simulink model "Q3n"  (R2018a)
settings: Solver=FixedStepDiscrete  StartTime=0.0  StopTime=0.42  RelTol=1e-3
libraries: powerlib x14, powerlib_meascontrol x3, dspstat3 x2, pePowerMeasurement x1
settings Model: Creator=hakkı  LastModifiedBy=hakkı

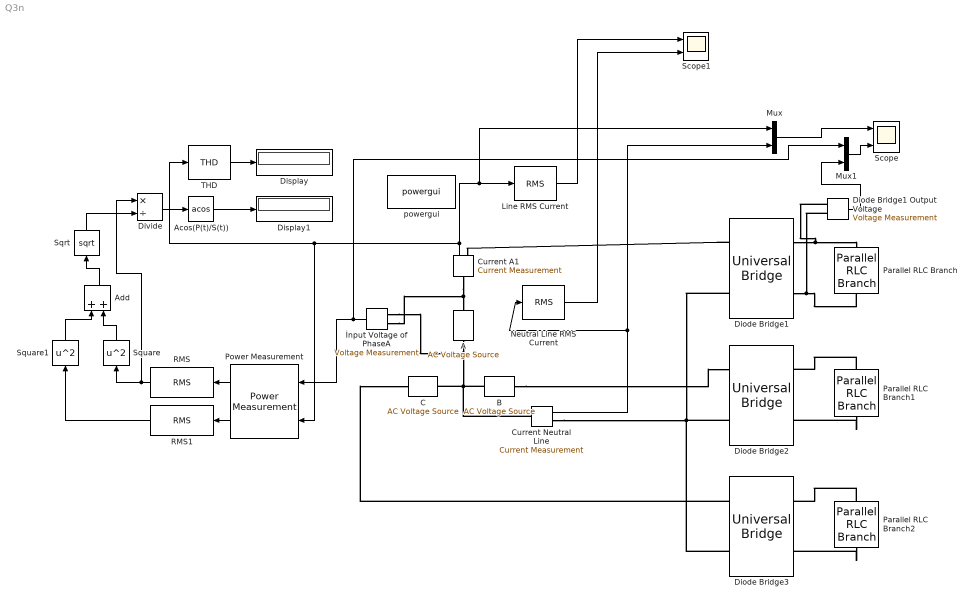
== system Q3n ==
  " İnput Voltage of PhaseA " : powerlib/Measurements/Voltage Measurement  PhasorSimulation=off  OutputType=Complex  PSBequivalent=0
  A : powerlib/Electrical Sources/AC Voltage Source  Amplitude=326.5986323710904130929712099607855189287929974208893504576  Phase=0  Frequency=50  SampleTime=0  Measurements=None  BusType=swing  Pref=10e3  Qref=0  Qmin=-inf  Qmax=+inf
  Acos(P(t)/S(t)) : Trigonometry  Operator=acos
  Add : Sum
  B : powerlib/Electrical Sources/AC Voltage Source  Amplitude=326.5986323710904130929712099607855189287929974208893504576  Phase=120  Frequency=50  SampleTime=0  Measurements=None  BusType=swing  Pref=10e3  Qref=0  Qmin=-inf  Qmax=+inf
  C : powerlib/Electrical Sources/AC Voltage Source  Amplitude=326.5986323710904130929712099607855189287929974208893504576  Phase=240  Frequency=50  SampleTime=0  Measurements=None  BusType=swing  Pref=10e3  Qref=0  Qmin=-inf  Qmax=+inf
  Current A1 : powerlib/Measurements/Current Measurement  PhasorSimulation=off  OutputType=Complex  PSBequivalent=0
  Current Neutral Line : powerlib/Measurements/Current Measurement  PhasorSimulation=off  OutputType=Complex  PSBequivalent=0
  Diode Bridge1 : powerlib/Power Electronics/Universal Bridge  Arms=2  SnubberResistance=1e5  SnubberCapacitance=inf  Device=Diodes  Ron=1e-3  Lon=0  ForwardVoltages="[  0  0  ]"  ForwardVoltage=0  GTOparameters=[ 10e-6 , 20e-6 ]  IGBTparameters=[ 1e-6 , 2e-6 ]  Measurements=None  Measurements_2=None  converterType=Rectifier
  "Diode Bridge1 Output Voltage " : powerlib/Measurements/Voltage Measurement  PhasorSimulation=off  OutputType=Complex  PSBequivalent=0
  Diode Bridge2 : powerlib/Power Electronics/Universal Bridge  Arms=2  SnubberResistance=1e5  SnubberCapacitance=inf  Device=Diodes  Ron=1e-3  Lon=0  ForwardVoltages="[  0  0  ]"  ForwardVoltage=0  GTOparameters=[ 10e-6 , 20e-6 ]  IGBTparameters=[ 1e-6 , 2e-6 ]  Measurements=None  Measurements_2=None  converterType=Rectifier
  Diode Bridge3 : powerlib/Power Electronics/Universal Bridge  Arms=2  SnubberResistance=1e5  SnubberCapacitance=inf  Device=Diodes  Ron=1e-3  Lon=0  ForwardVoltages="[  0  0  ]"  ForwardVoltage=0  GTOparameters=[ 10e-6 , 20e-6 ]  IGBTparameters=[ 1e-6 , 2e-6 ]  Measurements=None  Measurements_2=None  converterType=Rectifier
  Display : Display
  Display1 : Display
  Divide : Product  Inputs=*/
  "Line RMS Current " : powerlib_meascontrol/Measurements/RMS  TrueRMS=on  Freq=50  RMSInit=0  Ts=1e-6
  Mux : Mux  Inputs=2
  Mux1 : Mux  Inputs=2
  Neutral Line RMS Current : powerlib_meascontrol/Measurements/RMS  TrueRMS=on  Freq=50  RMSInit=0  Ts=1e-6
  Parallel RLC Branch : powerlib/Elements/Parallel RLC Branch  LConnTagsString=a  RConnTagsString=__new0  BranchType=RC  Resistance=200  Inductance=1e-3  SetiL0=off  InitialCurrent=0  Capacitance=470e-6  Setx0=off  InitialVoltage=0  Measurements=None
  Parallel RLC Branch1 : powerlib/Elements/Parallel RLC Branch  LConnTagsString=a  RConnTagsString=__new0  BranchType=RC  Resistance=200  Inductance=1e-3  SetiL0=off  InitialCurrent=0  Capacitance=470e-6  Setx0=off  InitialVoltage=0  Measurements=None
  Parallel RLC Branch2 : powerlib/Elements/Parallel RLC Branch  LConnTagsString=a  RConnTagsString=__new0  BranchType=RC  Resistance=200  Inductance=1e-3  SetiL0=off  InitialCurrent=0  Capacitance=470e-6  Setx0=off  InitialVoltage=0  Measurements=None
  Power Measurement : pePowerMeasurement/Power Measurement  OverrideUsingVariant=Discrete  F=50  K=[0 1 2 3]  Ts=1e-06
  RMS : dspstat3/RMS  run=off  directionMode=Each column  dimension=1  InputProcessing=Columns as channels (frame based)  reset_popup=None
  RMS1 : dspstat3/RMS  run=off  directionMode=Each column  dimension=1  InputProcessing=Columns as channels (frame based)  reset_popup=None
  Scope : Scope  NumInputPorts=2
  Scope1 : Scope  NumInputPorts=2
  Sqrt : Sqrt  SaturateOnIntegerOverflow=on
  Square : Math  Operator=square  SaturateOnIntegerOverflow=on
  Square1 : Math  Operator=square  SaturateOnIntegerOverflow=on
  THD : powerlib_meascontrol/Measurements/THD  Freq=50  Ts=1e-6
  powergui : powerlib/powergui  Priority=1  SimulationMode=Discrete  SampleTime=1e-6  frequency=60  Iterations=50  frequencyindice=50  Pbase=100e6  ErrMax=1e-4  UnitsV=kV  UnitsW=MW  buscounter=0  FunctionMessages=off  echomessages=off  EnableUseOfTLC=off  CurrentSourceSwitches=off  DisableSnubberDevices=off  DisableRonSwitches=off  DisableVfSwitches=off  DisplayEquations=off  SolverType=Tustin/Backward Euler (TBE)  Interpol=off  ExternalGateDelay=off  methode=off  Ts=100  x0status=blocks  SPID=on  SwTol=0  HookPort=off  RestoreLinks=warning  ResistiveCurrentMeasurement=off  Frange=[0:2:500]  Ylog=off  Xlog=on  ShowGrid=off  save=off  variable=ZData  structure=0  ZoomFFT=off  StartTime=0.0  cycles=1  DisplayStyle=1  fundamental=60  FreqAxis=off  MaxFrequency=1000  frequencyindicesteady=1  RmsSteady=1  display=off
  wires:
  Current A1/1 -> THD/1, Power Measurement/2, Mux/1, "Line RMS Current "/1
  " İnput Voltage of PhaseA "/1 -> Mux1/1, Power Measurement/1
  Square1/1 -> Add/1
  Add/1 -> Sqrt/1
  Sqrt/1 -> Divide/2
  Divide/1 -> Acos(P(t)/S(t))/1
  Square/1 -> Add/2
  Power Measurement/1 -> RMS/1
  RMS/1 -> Divide/1, Square/1
  Power Measurement/2 -> RMS1/1
  RMS1/1 -> Square1/1
  THD/1 -> Display/1
  Acos(P(t)/S(t))/1 -> Display1/1
  Mux/1 -> Scope/1
  Current Neutral Line/1 -> Neutral Line RMS Current/1, Mux/2
  Neutral Line RMS Current/1 -> Scope1/2
  "Line RMS Current "/1 -> Scope1/1
  "Diode Bridge1 Output Voltage "/1 -> Mux1/2
  Mux1/1 -> Scope/2
  connections:
  A/LConn1 -- " İnput Voltage of PhaseA "/LConn2 -- Current Neutral Line/LConn1 -- B/LConn1 -- C/LConn1
  Diode Bridge1/RConn1 -- "Diode Bridge1 Output Voltage "/LConn1 -- Parallel RLC Branch/LConn1
  Diode Bridge1/RConn2 -- "Diode Bridge1 Output Voltage "/LConn2 -- Parallel RLC Branch/RConn1
  Parallel RLC Branch1/RConn1 -- Diode Bridge2/RConn2
  Parallel RLC Branch1/LConn1 -- Diode Bridge2/RConn1
  Parallel RLC Branch2/LConn1 -- Diode Bridge3/RConn1
  Parallel RLC Branch2/RConn1 -- Diode Bridge3/RConn2
  Current A1/LConn1 -- " İnput Voltage of PhaseA "/LConn1 -- A/RConn1
  Diode Bridge3/LConn2 -- Current Neutral Line/RConn1 -- Diode Bridge1/LConn2 -- Diode Bridge2/LConn2
  Diode Bridge1/LConn1 -- Current A1/RConn1
  B/RConn1 -- Diode Bridge2/LConn1
  Diode Bridge3/LConn1 -- C/RConn1
